simulink model "inverter_npc_svpwm"  (R2019b)
settings: Solver=FixedStepAuto  StartTime=0.0  StopTime=0.1  FixedStep=To  RelTol=1e-3
PreLoadFcn:
  | clear;
  | run('m_svpwm_npc.m');
values from neighbouring files (symbols this model uses):
  Amp = 1    [m_svpwm_npc.m]
  Cf = 25e-6    (= 2.5e-05)    [m_svpwm_npc.m]
  Lf = 0.1e-3    (= 0.0001)    [m_svpwm_npc.m]
  To = Ts/1000    (= 5e-08)    [m_svpwm_npc.m]
  Ts = 1/Fs    (= 5e-05)    [m_svpwm_npc.m]
libraries: powerlib x19, simulink x6, simulink_extras x1, powerlib_meascontrol x1
settings Model: Creator=Dmitry  LastModifiedBy=NPT

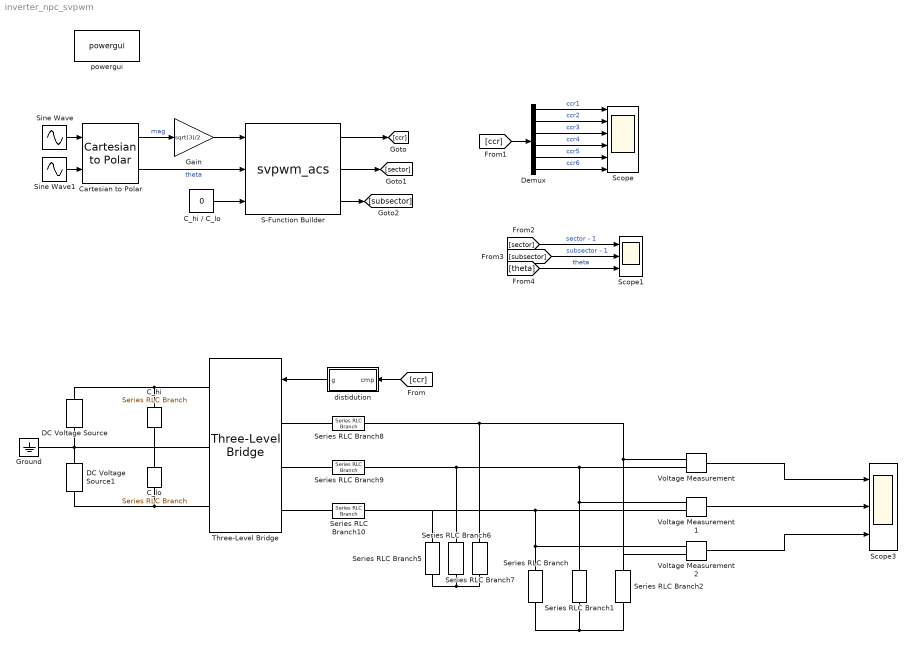
== system inverter_npc_svpwm ==
  C_hi : powerlib/Elements/Series RLC Branch  LConnTagsString=__new0  RConnTagsString=__new0  BranchType=RC  Resistance=0.001  Inductance=1e-3  SetiL0=off  InitialCurrent=0  Capacitance=1e-6  Setx0=off  InitialVoltage=0  Measurements=None
      settings: SourceProductName=Simscape Electrical
  C_hi / C_lo : Constant  Value=0
  C_lo : powerlib/Elements/Series RLC Branch  LConnTagsString=__new0  RConnTagsString=__new0  BranchType=RC  Resistance=0.001  Inductance=1e-3  SetiL0=off  InitialCurrent=0  Capacitance=1e-6  Setx0=off  InitialVoltage=0  Measurements=None
      settings: SourceProductName=Simscape Electrical
  Cartesian to Polar : simulink_extras/Transformations/Cartesian to Polar
      settings: SourceProductName=Simulink
  DC Voltage Source : powerlib/Electrical Sources/DC Voltage Source  Amplitude=350  Measurements=None
      settings: SourceProductName=Simscape Electrical
  DC Voltage Source1 : powerlib/Electrical Sources/DC Voltage Source  Amplitude=350  Measurements=None
      settings: SourceProductName=Simscape Electrical
  Demux : Demux  Outputs=6
  Gain : Gain  Gain=sqrt(3)/2
  Ground : powerlib/Elements/Ground  LConnTagsString=a
      settings: SourceProductName=Simscape Electrical
  S-Function Builder : S-Function  InitFcn=try, set_param(gcb,'FunctionName','svpwm_acs'), end  FunctionName=svpwm_acs  Parameters=Ts  SFunctionModules=svpwm_acs_wrapper CSVPWM_NPC  SFunctionDeploymentMode=off  EnableBusSupport=off  mask(S-Function Builder){}
      mask help: Simulink:masks:SFunctionBuilder_MD
      mask init:
      | val = [[.9  0.75 0.75 1 1 .9 .9 1]',[1 1 0.75 0.75 .9 .9 1 .9]'];try , sys = get_param(gcb,'SfunBuilderFcnName');if isempty(sys), sys = get_param(gcb,'FunctionName'); end,catch, sys = get_param(gcb,'FunctionName'); end
      settings: CopyFcn=set_param(gcbh,'LinkStatus','none')  PreSaveFcn=try, set_param(gcb,'FunctionName','svpwm_acs'), end  OpenFcn=sfunctionwizard(gcbh)
      mask Display: plot(val(:,1),val(:,2)),disp(sys), port_label('input',1,'mag'), port_label('input',2,'th'), port_label('input',3,'selCap'), port_label('output',1,'ccr'), port_label('output',2,'sctr'), port_label('output',3,'subsctr')
  Scope : Scope  NumInputPorts=6
  Scope1 : Scope  NumInputPorts=3
  Scope3 : Scope  NumInputPorts=3
  Series RLC Branch : powerlib/Elements/Series RLC Branch  LConnTagsString=__new0  RConnTagsString=__new0  BranchType=R  Resistance=10  Inductance=1e-3  SetiL0=off  InitialCurrent=0  Capacitance=1e-6  Setx0=off  InitialVoltage=0  Measurements=None
      settings: SourceProductName=Simscape Electrical
  Series RLC Branch1 : powerlib/Elements/Series RLC Branch  LConnTagsString=__new0  RConnTagsString=__new0  BranchType=R  Resistance=10  Inductance=1e-3  SetiL0=off  InitialCurrent=0  Capacitance=1e-6  Setx0=off  InitialVoltage=0  Measurements=None
      settings: SourceProductName=Simscape Electrical
  Series RLC Branch10 : powerlib/Elements/Series RLC Branch  LConnTagsString=__new0  RConnTagsString=__new0  BranchType=L  Resistance=10  Inductance=Lf  SetiL0=off  InitialCurrent=0  Capacitance=1e-6  Setx0=off  InitialVoltage=0  Measurements=None
      settings: SourceProductName=Simscape Electrical
  Series RLC Branch2 : powerlib/Elements/Series RLC Branch  LConnTagsString=__new0  RConnTagsString=__new0  BranchType=R  Resistance=10  Inductance=1e-3  SetiL0=off  InitialCurrent=0  Capacitance=1e-6  Setx0=off  InitialVoltage=0  Measurements=None
      settings: SourceProductName=Simscape Electrical
  Series RLC Branch5 : powerlib/Elements/Series RLC Branch  LConnTagsString=__new0  RConnTagsString=__new0  BranchType=C  Resistance=1000  Inductance=1e-3  SetiL0=off  InitialCurrent=0  Capacitance=Cf  Setx0=off  InitialVoltage=0  Measurements=None
      settings: SourceProductName=Simscape Electrical
  Series RLC Branch6 : powerlib/Elements/Series RLC Branch  LConnTagsString=__new0  RConnTagsString=__new0  BranchType=C  Resistance=1000  Inductance=1e-3  SetiL0=off  InitialCurrent=0  Capacitance=Cf  Setx0=off  InitialVoltage=0  Measurements=None
      settings: SourceProductName=Simscape Electrical
  Series RLC Branch7 : powerlib/Elements/Series RLC Branch  LConnTagsString=__new0  RConnTagsString=__new0  BranchType=C  Resistance=1000  Inductance=1e-3  SetiL0=off  InitialCurrent=0  Capacitance=Cf  Setx0=off  InitialVoltage=0  Measurements=None
      settings: SourceProductName=Simscape Electrical
  Series RLC Branch8 : powerlib/Elements/Series RLC Branch  LConnTagsString=__new0  RConnTagsString=__new0  BranchType=L  Resistance=10  Inductance=Lf  SetiL0=off  InitialCurrent=0  Capacitance=1e-6  Setx0=off  InitialVoltage=0  Measurements=None
      settings: SourceProductName=Simscape Electrical
  Series RLC Branch9 : powerlib/Elements/Series RLC Branch  LConnTagsString=__new0  RConnTagsString=__new0  BranchType=L  Resistance=10  Inductance=Lf  SetiL0=off  InitialCurrent=0  Capacitance=1e-6  Setx0=off  InitialVoltage=0  Measurements=None
      settings: SourceProductName=Simscape Electrical
  Sine Wave : Sin  Amplitude=Amp  Frequency=100*pi  Phase=pi/2  SampleTime=Ts
  Sine Wave1 : Sin  Amplitude=Amp  Frequency=100*pi  SampleTime=Ts
  Three-Level Bridge : powerlib/Power Electronics/Three-Level Bridge  Arms=3  SnubberResistance=1e5  SbubberCapacitance=inf  Device=IGBT / Diodes  Ron=1e-3  ForwardVoltages="[  0  0  ]"  Measurements=None
      settings: SourceProductName=Simscape Electrical  SourceProductBaseCode=PS
  Voltage Measurement : powerlib/Measurements/Voltage Measurement  PhasorSimulation=off  OutputType=Complex  PSBequivalent=0
      settings: SourceProductName=Simscape Electrical
  Voltage Measurement1 : powerlib/Measurements/Voltage Measurement  PhasorSimulation=off  OutputType=Complex  PSBequivalent=0
      settings: SourceProductName=Simscape Electrical
  Voltage Measurement2 : powerlib/Measurements/Voltage Measurement  PhasorSimulation=off  OutputType=Complex  PSBequivalent=0
      settings: SourceProductName=Simscape Electrical
  distidution : Subsystem
  powergui : powerlib/powergui  Priority=1  SimulationMode=Discrete  SampleTime=To  frequency=60  Iterations=50  frequencyindice=0  Pbase=100e6  ErrMax=1e-4  UnitsV=kV  UnitsW=MW  buscounter=0  FunctionMessages=off  echomessages=off  EnableUseOfTLC=off  CurrentSourceSwitches=off  DisableSnubberDevices=off  DisableRonSwitches=off  DisableVfSwitches=off  DisplayEquations=off  AutomaticDiscreteSolvers=off  SolverType=Tustin/Backward Euler (TBE)  Interpol=off  ExternalGateDelay=off  methode=off  Ts=100  x0status=blocks  SPID=on  SwTol=0  HookPort=off  NonlinearTolerance=1e-4  nMaxIteration=100  ContinueOnMaxIteration=off  RestoreLinks=warning  ResistiveCurrentMeasurement=off  Frange=[0:2:500]  Ylog=off  Xlog=on  ShowGrid=off  save=off  variable=ZData  structure=0  ZoomFFT=off  StartTime=0.0  cycles=1  DisplayStyle=1  fundamental=60  FreqAxis=off  MaxFrequency=1000  frequencyindicesteady=1  RmsSteady=1  display=off
      settings: SourceProductName=Simscape Electrical
  wires:
  Sine Wave/1 -> Cartesian to Polar/1
  Sine Wave1/1 -> Cartesian to Polar/2
  Cartesian to Polar/1 -> Gain/1  "mag"
  Cartesian to Polar/2 -> S-Function Builder/2  "theta"
  C_hi / C_lo/1 -> S-Function Builder/3
  Demux/1 -> Scope/1  "ccr1"
  Demux/2 -> Scope/2  "ccr2"
  Demux/3 -> Scope/3  "ccr3"
  Demux/4 -> Scope/4  "ccr4"
  Demux/5 -> Scope/5  "ccr5"
  Demux/6 -> Scope/6  "ccr6"
  S-Function Builder/2 -> [sector]
  S-Function Builder/3 -> [subsector]
  Gain/1 -> S-Function Builder/1
  distidution/1(g) -> Three-Level Bridge/1
  Voltage Measurement/1 -> Scope3/1
  Voltage Measurement1/1 -> Scope3/2
  Voltage Measurement2/1 -> Scope3/3
  S-Function Builder/1 -> [ccr]
  [ccr] -> distidution/1(cmp)
  [ccr] -> Demux/1
  [sector] -> Scope1/1  "sector - 1"
  [subsector] -> Scope1/2  "subsector - 1"
  [theta] -> Scope1/3  "theta"
  connections:
  DC Voltage Source1/RConn1 -- Ground/LConn1 -- C_lo/LConn1 -- C_hi/RConn1 -- Three-Level Bridge/RConn2 -- DC Voltage Source/LConn1
  Three-Level Bridge/RConn1 -- C_hi/LConn1 -- DC Voltage Source/RConn1
  Three-Level Bridge/RConn3 -- C_lo/RConn1 -- DC Voltage Source1/LConn1
  Series RLC Branch/RConn1 -- Series RLC Branch2/RConn1 -- Series RLC Branch1/RConn1
  Series RLC Branch5/RConn1 -- Series RLC Branch6/RConn1 -- Series RLC Branch7/RConn1
  Series RLC Branch1/LConn1 -- Voltage Measurement1/LConn1 -- Series RLC Branch6/LConn1 -- Series RLC Branch9/RConn1 -- Voltage Measurement/LConn2
  Voltage Measurement2/LConn1 -- Series RLC Branch5/LConn1 -- Series RLC Branch10/RConn1 -- Voltage Measurement1/LConn2 -- Series RLC Branch/LConn1
  Series RLC Branch8/LConn1 -- Three-Level Bridge/LConn1
  Voltage Measurement/LConn1 -- Series RLC Branch2/LConn1 -- Voltage Measurement2/LConn2 -- Series RLC Branch7/LConn1 -- Series RLC Branch8/RConn1
  Series RLC Branch9/LConn1 -- Three-Level Bridge/LConn2
  Three-Level Bridge/LConn3 -- Series RLC Branch10/LConn1

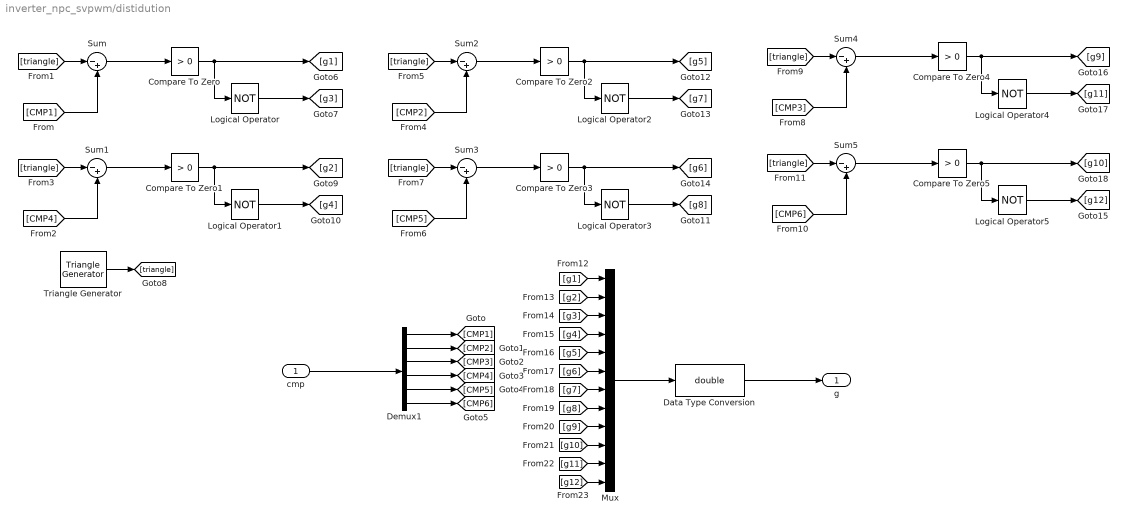
== system inverter_npc_svpwm/distidution ==
  cmp : Inport
  Compare To Zero{,1..5} (6 alike) : simulink/Logic and Bit Operations/Compare To Zero  relop=>  OutDataTypeStr=boolean
  Data Type Conversion : DataTypeConversion  OutDataTypeStr=double
  Demux1 : Demux  Outputs=6
  Logical Operator{,1..5} (6 alike) : Logic  Operator=NOT  AllPortsSameDT=off  OutDataTypeStr=boolean
  Mux : Mux  Inputs=12
  Sum{,1..5} (6 alike) : Sum  Inputs=|-+
  Triangle Generator : powerlib_meascontrol/Pulse & Signal Generators/Triangle Generator  Freq=Fs  Phase=0  Ts=To
      settings: SourceProductName=Simscape Electrical
  g : Outport
  wires:
  cmp/1 -> Demux1/1
  Demux1/1 -> [CMP1]
  Demux1/2 -> [CMP2]
  Demux1/3 -> [CMP3]
  Demux1/4 -> [CMP4]
  Demux1/5 -> [CMP5]
  Demux1/6 -> [CMP6]
  [CMP1] -> Sum/2
  Compare To Zero/1 -> [g1], Logical Operator/1
  Logical Operator/1 -> [g3]
  Triangle Generator/1 -> [triangle]
  [triangle] -> Sum/1
  [triangle] -> Sum1/1
  Logical Operator1/1 -> [g4]
  Compare To Zero1/1 -> Logical Operator1/1, [g2]
  [CMP4] -> Sum1/2
  [CMP5] -> Sum3/2
  Compare To Zero3/1 -> [g6], Logical Operator3/1
  Logical Operator3/1 -> [g8]
  [triangle] -> Sum3/1
  [triangle] -> Sum2/1
  Logical Operator2/1 -> [g7]
  Compare To Zero2/1 -> Logical Operator2/1, [g5]
  [CMP2] -> Sum2/2
  [CMP3] -> Sum4/2
  Compare To Zero4/1 -> [g9], Logical Operator4/1
  Logical Operator4/1 -> [g11]
  [triangle] -> Sum4/1
  [triangle] -> Sum5/1
  Logical Operator5/1 -> [g12]
  Compare To Zero5/1 -> Logical Operator5/1, [g10]
  [CMP6] -> Sum5/2
  Mux/1 -> Data Type Conversion/1
  [g1] -> Mux/1
  [g2] -> Mux/2
  [g3] -> Mux/3
  [g4] -> Mux/4
  [g5] -> Mux/5
  [g6] -> Mux/6
  [g7] -> Mux/7
  [g8] -> Mux/8
  [g9] -> Mux/9
  [g10] -> Mux/10
  [g11] -> Mux/11
  [g12] -> Mux/12
  Data Type Conversion/1 -> g/1
  Sum/1 -> Compare To Zero/1
  Sum1/1 -> Compare To Zero1/1
  Sum2/1 -> Compare To Zero2/1
  Sum3/1 -> Compare To Zero3/1
  Sum4/1 -> Compare To Zero4/1
  Sum5/1 -> Compare To Zero5/1
